simulink model "FW_LinLateralModel"  (R2015a)
settings: Solver=ode45  StartTime=0.0  StopTime=Trun  RelTol=1e-3
undefined symbols (not defined in the file): Initial_Lat, Initial_Lat_Roll, Ldel_a, Ldel_r, Lp, Lr, Lv, Ndel_a, Ndel_r, Np, Nr, Nv, Tr_p, Tr_phi, Tr_q, Tr_r, Tr_theta, Ydel_a, Ydel_r, Yp, Yr, Yv
settings Model: Creator=user  LastModifiedBy=user

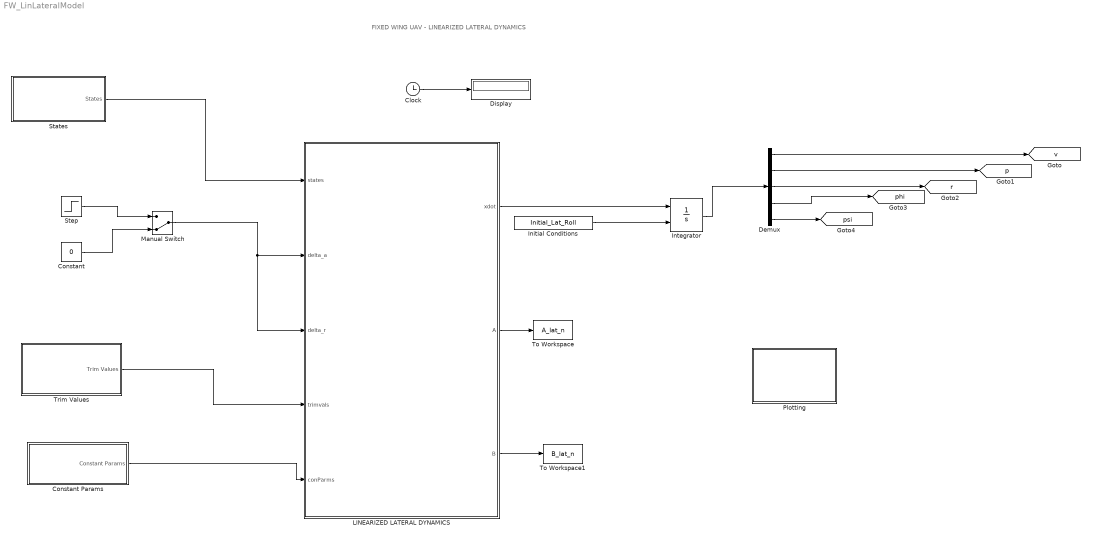
== system FW_LinLateralModel ==
  note: FIXED WING UAV - LINEARIZED LATERAL DYNAMICS
  Clock : Clock
  Constant : Constant  Value=0
  Constant Params : Subsystem
  Demux : Demux  Outputs=5
  Display : Display
  Initial Conditions : Constant  Value=Initial_Lat_Roll
  Integrator : Integrator  InitialConditionSource=external  InitialCondition=Initial_Lat
  LINEARIZED LATERAL DYNAMICS : MATLAB Function  TreatAsAtomicUnit=on
  Manual Switch : ManualSwitch  CurrentSetting=0
  Plotting : Subsystem
  States : Subsystem
  Step : Step  SampleTime=0
  To Workspace : ToWorkspace  VariableName=A_lat_n  SampleTime=-1
      settings: MaxDataPoints=1
  To Workspace1 : ToWorkspace  VariableName=B_lat_n  SampleTime=-1
      settings: MaxDataPoints=1
  Trim Values : Subsystem
  tag scope: p=global, phi=global, psi=global, r=global, v=global
  wires:
  LINEARIZED LATERAL DYNAMICS/1(xdot) -> Integrator/1
  LINEARIZED LATERAL DYNAMICS/3(B) -> To Workspace1/1
  Integrator/1 -> Demux/1
  Demux/1 -> [v]
  Demux/2 -> [p]
  Demux/3 -> [r]
  Demux/4 -> [phi]
  Demux/5 -> [psi]
  States/1(States) -> LINEARIZED LATERAL DYNAMICS/1(states)
  LINEARIZED LATERAL DYNAMICS/2(A) -> To Workspace/1
  Trim Values/1(Trim Values) -> LINEARIZED LATERAL DYNAMICS/4(trimvals)
  Constant Params/1("Constant Params ") -> LINEARIZED LATERAL DYNAMICS/5(conParms)
  Clock/1 -> Display/1
  Step/1 -> Manual Switch/1
  Constant/1 -> Manual Switch/2
  Manual Switch/1 -> LINEARIZED LATERAL DYNAMICS/3(delta_r), LINEARIZED LATERAL DYNAMICS/2(delta_a)
  Initial Conditions/1 -> Integrator/2

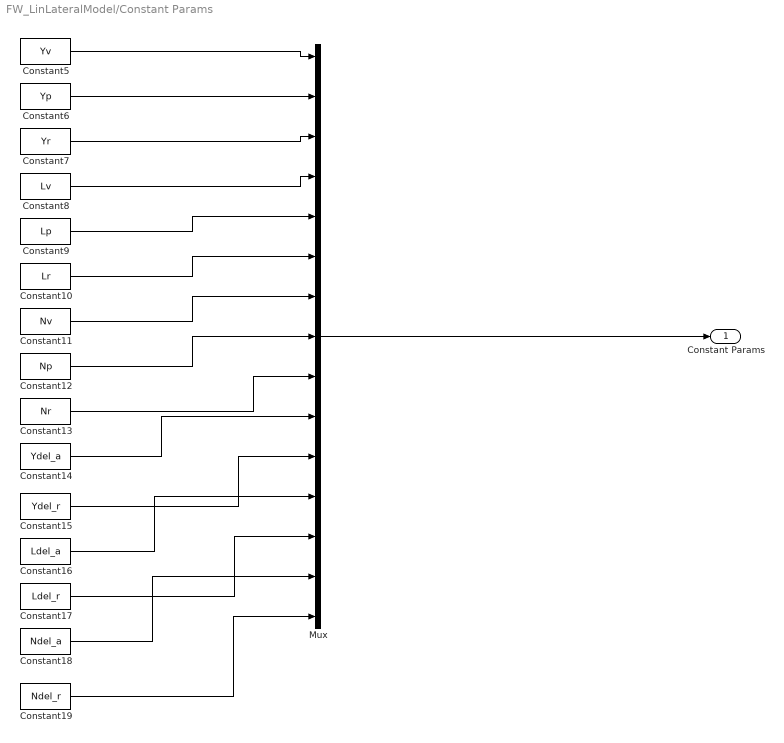
== system FW_LinLateralModel/Constant Params ==
  Constant10 : Constant  Value=Lr
  Constant11 : Constant  Value=Nv
  Constant12 : Constant  Value=Np
  Constant13 : Constant  Value=Nr
  Constant14 : Constant  Value=Ydel_a
  Constant15 : Constant  Value=Ydel_r
  Constant16 : Constant  Value=Ldel_a
  Constant17 : Constant  Value=Ldel_r
  Constant18 : Constant  Value=Ndel_a
  Constant19 : Constant  Value=Ndel_r
  Constant5 : Constant  Value=Yv
  Constant6 : Constant  Value=Yp
  Constant7 : Constant  Value=Yr
  Constant8 : Constant  Value=Lv
  Constant9 : Constant  Value=Lp
  Mux : Mux  Inputs=15
  "Constant Params " : Outport
  wires:
  Constant14/1 -> Mux/10
  Constant15/1 -> Mux/11
  Constant19/1 -> Mux/15
  Constant17/1 -> Mux/13
  Constant18/1 -> Mux/14
  Constant16/1 -> Mux/12
  Constant6/1 -> Mux/2
  Constant5/1 -> Mux/1
  Constant7/1 -> Mux/3
  Constant13/1 -> Mux/9
  Constant10/1 -> Mux/6
  Constant8/1 -> Mux/4
  Constant9/1 -> Mux/5
  Constant11/1 -> Mux/7
  Constant12/1 -> Mux/8
  Mux/1 -> "Constant Params "/1

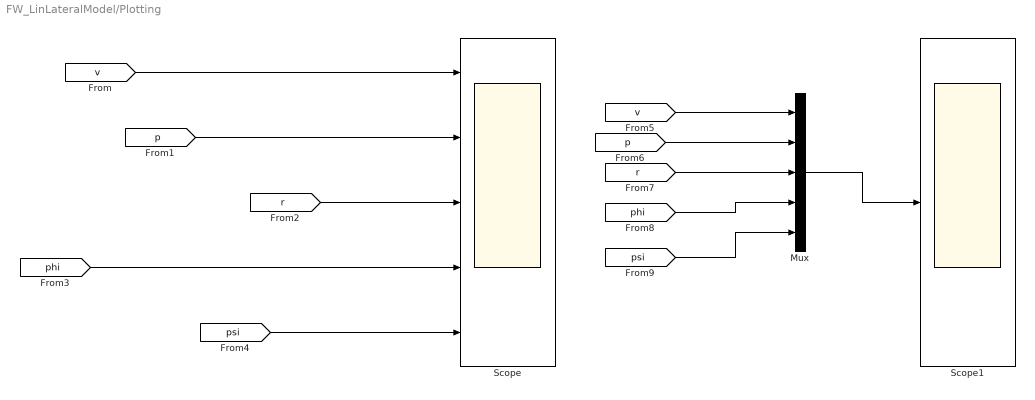
== system FW_LinLateralModel/Plotting ==
  Mux : Mux  Inputs=5
  Scope : Scope  NumInputPorts=5
      settings: YMin=-5~-5~-5~-5~-5  YMax=5~5~5~5~5
  Scope1 : Scope
      settings: ShowLegends=on
  wires:
  [phi] -> Scope/4
  [p] -> Scope/2
  [psi] -> Scope/5
  [v] -> Scope/1
  [r] -> Scope/3
  [v] -> Mux/1
  [p] -> Mux/2
  [r] -> Mux/3
  [phi] -> Mux/4
  [psi] -> Mux/5
  Mux/1 -> Scope1/1

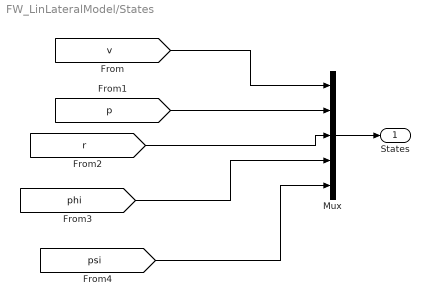
== system FW_LinLateralModel/States ==
  Mux : Mux  Inputs=5
  States : Outport  PortDimensions=5
  wires:
  [r] -> Mux/3
  [phi] -> Mux/4
  [psi] -> Mux/5
  Mux/1 -> States/1
  [v] -> Mux/1
  [p] -> Mux/2

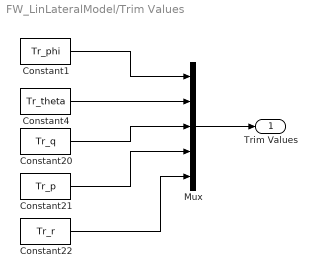
== system FW_LinLateralModel/Trim Values ==
  Constant1 : Constant  Value=Tr_phi
  Constant20 : Constant  Value=Tr_q
  Constant21 : Constant  Value=Tr_p
  Constant22 : Constant  Value=Tr_r
  Constant4 : Constant  Value=Tr_theta
  Mux : Mux  Inputs=5
  Trim Values : Outport  PortDimensions=5
  wires:
  Constant4/1 -> Mux/2
  Mux/1 -> Trim Values/1
  Constant1/1 -> Mux/1
  Constant21/1 -> Mux/4
  Constant20/1 -> Mux/3
  Constant22/1 -> Mux/5

== matlab function FW_LinLateralModel/LINEARIZED LATERAL DYNAMICS ==
  data: states input; xdot output; delta_a input; delta_r input; A output; B output; trimvals input; conParms input
function [xdot,A,B] = Linearized_Lateral_Dynamics(states,delta_a,delta_r,trimvals,conParms)
%% LINEARIZED LATERAL DYNAMICS
% States: [v,p,r,phi,psi]
% Inputs:  [del_a,del_r]
% Paramters used
% P : Paramters of the system
% Tr : Trim Values
P_gravity = 9.81;
%% States
v = states(1);
p =states(2);
r = states(3);
phi =states(4);
psi = states(5);
%% Trim Values
Tr_phi = trimvals(1);
Tr_theta=trimvals(2);
Tr_q=trimvals(3);
Tr_p=trimvals(4);
Tr_r=trimvals(5);
%% Constant Parameter
Yv=conParms(1);
Yp=conParms(2);
Yr=conParms(3);
Lv=conParms(4);
Lp=conParms(5);
Lr=conParms(6);
Nv=conParms(7);
Np=conParms(8);
Nr=conParms(9);
Ydel_a=conParms(10);
Ydel_r=conParms(11);
Ldel_a=conParms(12);
Ldel_r=conParms(13);
Ndel_a=conParms(14);
Ndel_r=conParms(15);
%---------------------------------------
%  State Space Matrices
A = [Yv Yp Yr P_gravity*cos(Tr_theta)*cos(Tr_phi) 0;
     Lv Lp Lr 0 0;
     Nv Np Nr 0 0;
     0 1 cos(Tr_phi)*tan(Tr_theta) Tr_q*cos(Tr_phi)*tan(Tr_theta)-Tr_r*sin(Tr_phi)*tan(Tr_theta) 0;
     0 0 cos(Tr_phi)*sec(Tr_theta) Tr_p*cos(Tr_phi)*sec(Tr_theta)-Tr_r*sin(Tr_phi)*sec(Tr_theta) 0];
 
B  = [Ydel_a Ydel_r; 
      Ldel_a Ldel_r;
      Ndel_a Ndel_r;
      0 0;
      0 0];

x = [v;p;r;phi;psi];
u = [delta_a;delta_r];

xdot = A*x + B*u;


% Lateral State Space Model
